simulink library "GOcontroll_Moduline_Target"  (R2023b)
settings: Solver=ode45  StartTime=0.0  StopTime=10.0  RelTol=1e-3  EnableMultiTasking=on
PreLoadFcn:
  | compile_gocontroll_mex;
values from neighbouring files (symbols this model uses):
  id = 2    [sfcn_UDPReceive.m]    (also in sfcn_UDPSend.m = 4)
undefined symbols (not defined in the file or in its folder): C_Cb1Pt10, Cb1Pt10_RAW_ERR_HIGH, Cb1Pt10_RAW_ERR_LOW, Cb1Pt10_SIG_ERR_HIGH, Cb1Pt10_SIG_ERR_LOW, Cb1Pt10_SIG_WAR_HIGH, Cb1Pt10_SIG_WAR_LOW, Pres_0_20_bar_500_4500_mv_inv, signal_x_RAW_ERR_HIGH, signal_x_RAW_ERR_LOW, signal_x_SIG_ERR_HIGH, signal_x_SIG_ERR_LOW, signal_x_SIG_WAR_HIGH, signal_x_SIG_WAR_LOW, signal_x_SPN, Valve1_ACTIVE_DUTY_CYCLE, Valve1_MAX_CURRENT, Valve1_MIN_CURRENT, Valve1_SPN
libraries: $bdroot x17, simulink x12, canmsglib x4
(part 3 of 5)

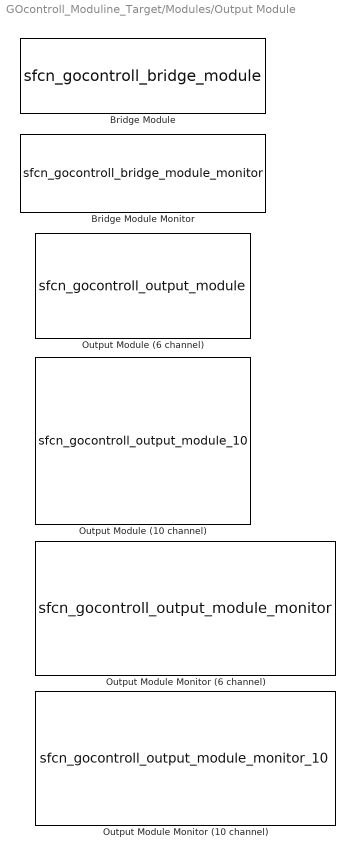
== system GOcontroll_Moduline_Target/Modules/Output Module ==
  Bridge Module : M-S-Function  FunctionName=sfcn_gocontroll_bridge_module  Parameters=tsamp  mask(Bridge Module){tsamp=1, ContrType=GOcontroll Moduline IV, moduleSlot=Moduleslot 1, C1func=Disable (output disabled), C1freq=100 Hz, C2func=Disable (output disabled), C2freq=100 Hz}
      mask prompts: tsamp "Sample time"; ContrType "Controller Type"; moduleSlot "Module Slot"; C1func "Function select"; C1freq "Frequency"; C2func "Function select"; C2freq "Frequency"
      mask help:
      | With this function block, you can configure each output of the bridge module (202001xx). During initialization of the controller, the corresponding outputs of the module are set according the settings. During runtime, the value pushed into the block will control the outputs.
      |
      | Module slot:
      | Sets the location of the module slot where the module is physically
      | plugged into.
      |
      | Channel tabs:
      | Each ouput has its own configuration tab.
      |
      | Function select:
      | Select the desired output configuration.
      |
      | Frequency:
      | In case a duty cycle is used, select the frequency.
      mask init:
      | % array with pinID infos
      | 	moduleSlotInfoStrings = {  	'Module Slot 1',  ...
      | 								'Module Slot 2',  ...
      | 								'Module Slot 3',  ...
      | 								'Module Slot 4',  ...
      | 								'Module Slot 5',  ...
      | 								'Module Slot 6',  ...
      | 								'Module Slot 7',  ...
      | 								'Module Slot 8'};
      | 	% construct the pinID info string
      | 	moduleSlotInfoStr = moduleSlotInfoStrings{moduleSlot};
      | 
      | 
      | 	if(moduleSlot == 1 || moduleSlot == 2)
      | 		connectorId = 'A';
      | 	elseif(moduleSlot == 3 || moduleSlot == 4)
      | 		connectorId = 'B';
      | 	elseif(moduleSlot == 5 || moduleSlot == 6)
      | 		connectorId = 'D';
      | 	else
      | 		connectorId = 'E';
      | 	end
      | 
      | 	if (ContrType == 1) % Moduline IV
      | 		if (mod(moduleSlot,2) == 1) %uneven
      | 			pin1Id = 'Pin 11,12,13';
      | 			pin2Id = 'Pin 17,18,19';
      | 		else
      | 			pin1Id = 'Pin 8,9,10';
      | 			pin2Id = 'Pin 14,15,16';
      | 		end
      | 	elseif(ContrType == 2 || ContrType == 3) % Moduline mini / Moduline display
      | 		if(mod(moduleSlot,2) == 1)
      | 			pin1Id = 'Pin 13,14,15';
      | 			pin2Id = 'Pin 21,22,23';
      | 		else
      | 			pin1Id = 'Pin 10,11,12';
      | 			pin2Id = 'Pin 18,19,20';
      | 		end
      |     end
      |     % register rtw data here because the WriteRTW callback doesn't update
      |     % properly
      |     % Create resource keywords to be reserved in resource database
      | 	modelRTWFields = 	struct('moduleSlot', int2str(moduleSlot),	'C1func', int2str(C1func),'C1freq', int2str(C1freq),...
      | 										'C2func', int2str(C2func),'C2freq', int2str(C2freq));
      | 
      | 	set_param(gcb, 'RTWdata', modelRTWFields);
      mask TypeOptions ContrType: GOcontroll Moduline IV | GOcontroll Moduline Mini | GOcontroll Moduline Display
      mask Callback ContrType:
      | msk = Simulink.Mask.get(gcb);
      | p = msk.getParameter('moduleSlot');
      | 
      | func = get_param(gcb,'ContrType');
      | 
      | if(func == "GOcontroll Moduline IV")
      |     p.TypeOptions = {'Moduleslot 1','Moduleslot 2','Moduleslot 3','Moduleslot 4',...
      |                     'Moduleslot 5','Moduleslot 6','Moduleslot 7','Moduleslot 8'};
      | elseif(func == "GOcontroll Moduline Mini")
      |     p.TypeOptions = {'Moduleslot 1','Moduleslot 2','Moduleslot 3','Moduleslot 4'};
      | elseif (func == "GOcontroll Moduline Display")
      |     p.TypeOptions = {'Moduleslot 1','Moduleslot 2'};
      | end
      mask TypeOptions moduleSlot: Moduleslot 1 | Moduleslot 2 | Moduleslot 3 | Moduleslot 4 | Moduleslot 5 | Moduleslot 6 | Moduleslot 7 | Moduleslot 8
      mask TypeOptions C1func: Disable (output disabled) | Half Bridge duty cycle controlled 0% - 100% duty cycle ( 0 - 1000) | Low side switch  duty cycle controlled 0% - 100% duty cycle (0 - 1000) | High side switch  duty cycle controlled 0% - 100% duty cycle (0 - 1000) | Low side switch On - Off (1-0) | High side switch On - Off (1-0)
      mask TypeOptions C1freq: 100 Hz | 200 Hz | 500 Hz | 1 kHz | 2 kHz | 5 kHz | 10 kHz
      mask TypeOptions C2func: Disable (output disabled) | Half Bridge duty cycle controlled 0% - 100% duty cycle ( 0 - 1000) | Low side switch  duty cycle controlled 0% - 100% duty cycle (0 - 1000) | High side switch  duty cycle controlled 0% - 100% duty cycle (0 - 1000) | Low side switch On - Off (1-0) | High side switch On - Off (1-0)
      mask TypeOptions C2freq: 100 Hz | 200 Hz | 500 Hz | 1 kHz | 2 kHz | 5 kHz | 10 kHz
      mask DialogControl Container4 Prompt: Output 1
      mask DialogControl Container5 Prompt: Output 2
      mask Display:
      | fprintf('Bridge Module\n%s\n\n Controller Connector: %s', moduleSlotInfoStr,connectorId);
      | port_label('input', 1, pin1Id);
      | port_label('input', 2, pin2Id);
      | text(2, 6, ert_linux_target_version());
  Bridge Module Monitor : M-S-Function  FunctionName=sfcn_gocontroll_bridge_module_monitor  Parameters=tsamp  mask(Bridge Module Monitor){tsamp=1, ContrType=GOcontroll Moduline IV, moduleSlot=Moduleslot 1}
      mask prompts: tsamp "Sample time"; ContrType "Controller Type"; moduleSlot "Module Slot"
      mask help:
      | With this function block, you can read parameters from the specified bridge module (202001xx). The block will provide some information about the module such as:
      |
      | Module temperature:
      | The temperature in degrees from the output module.
      |
      | Module ground shift
      | In case the ground connection of the module is poor, the power ground is shifted. The value gives the ground difference in mV and schould be beneath 50 mV
      |
      | Channel current
      | Current related output for each output channel
      mask init:
      | % array with pinID infos
      | 	moduleSlotInfoStrings = {  	'Module slot 1',  ...\
      | 								  'Module slot 2',  ...\
      | 								  'Module slot 3',  ...\
      | 								  'Module slot 4',  ...\
      | 								  'Module slot 5',  ...\
      | 								  'Module slot 6',  ...\
      | 								  'Module slot 7',  ...\
      | 								  'Module slot 8'};
      | 	% construct the pinID info string
      | 	moduleSlotInfoStr = moduleSlotInfoStrings{moduleSlot};
      | 
      | 	if(moduleSlot == 1 || moduleSlot == 2)
      | 		connectorId = 'A';
      | 	elseif(moduleSlot == 3 || moduleSlot == 4)
      | 		connectorId = 'B';
      | 	elseif(moduleSlot == 5 || moduleSlot == 6)
      | 		connectorId = 'D';
      | 	else
      | 		connectorId = 'E';
      | 	end
      | 
      | 	if(ContrType == 1) % Moduline IV
      | 		if(mod(moduleSlot,2) == 1)
      | 			pin1Id = 'Pin 11,12,13';
      | 			pin2Id = 'Pin 17,18,19';
      | 		else
      | 			pin1Id = 'Pin 8,9,10';
      | 			pin2Id = 'Pin 14,15,16';
      | 		end
      | 	elseif(ContrType == 2 || ContrType == 3) % Moduline mini / Moduline display
      | 		if(mod(moduleSlot,2) == 1)
      | 			pin1Id = 'Pin 13,14,15';
      | 			pin2Id = 'Pin 21,22,23';
      | 		else
      | 			pin1Id = 'Pin 10,11,12';
      | 			pin2Id = 'Pin 18,19,20';
      | 		end
      | 	end
      |     % update RTWdata to call WriteRTW again
      | 	modelRTWFields = 	struct('moduleSlot', int2str(moduleSlot));
      | 
      | 	set_param(gcb, 'RTWdata', modelRTWFields);
      mask TypeOptions ContrType: GOcontroll Moduline IV | GOcontroll Moduline Mini | GOcontroll Moduline Display
      mask Callback ContrType:
      | msk = Simulink.Mask.get(gcb);
      |     p = msk.getParameter('moduleSlot');
      |     func = get_param(gcb,'ContrType');
      |     if(func == "GOcontroll Moduline IV")
      |         p.TypeOptions = {'Moduleslot 1','Moduleslot 2','Moduleslot 3','Moduleslot 4',...
      |                         'Moduleslot 5','Moduleslot 6','Moduleslot 7','Moduleslot 8'};
      |     elseif (func == "GOcontroll Moduline Mini")
      |         p.TypeOptions = {'Moduleslot 1','Moduleslot 2','Moduleslot 3','Moduleslot 4'};
      |     elseif (func == "GOcontroll Moduline Display")
      |         p.TypeOptions = {'Moduleslot 1','Moduleslot 2'};
      |     end
      mask TypeOptions moduleSlot: Moduleslot 1 | Moduleslot 2 | Moduleslot 3 | Moduleslot 4 | Moduleslot 5 | Moduleslot 6 | Moduleslot 7 | Moduleslot 8
      mask Display:
      | fprintf('Bridge Module Monitor\n%s\n\n Controller Connector: %s', moduleSlotInfoStr,connectorId);
      | port_label('output', 1, 'Temperature');
      | port_label('output', 2, 'Groundshift');
      | port_label('output', 3, pin1Id);
      | port_label('output', 4, pin2Id);
      | text(2, 6, ert_linux_target_version());
  Output Module (10 channel) : M-S-Function  FunctionName=sfcn_gocontroll_output_module_10  Parameters=tsamp  mask(10 Channel Output Module){tsamp=0.1, ContrType=GOcontroll Moduline IV, moduleSlot=Moduleslot 1, C12freq=200 Hz, C1func=Disable (output disabled), C2func=Disable (output disabled), C34freq=200 Hz, C3func=Disable (output disabled), C4func=Disable (output disabled), C56freq=200 Hz, C5func=Disable (output disabled), C6func=Disable (output disabled), C78freq=200 Hz, C7func=Disable (output disabled), C8func=Disable (output disabled), C910freq=200 Hz, C9func=Disable (output disabled), C10func=Disable (output disabled)}
      mask prompts: tsamp "Sample time"; ContrType "Controller type"; moduleSlot "Module slot"; C12freq "Frequency"; C1func "Channel 1 function"; C2func "Channel 2 function"; C34freq "Frequency"; C3func "Channel 3 function"; C4func "Channel 4 function"; C56freq "Frequency"; C5func "Channel 5 function"; C6func "Channel 6 function"; C78freq "Frequency"; C7func "Channel 7 function"; C8func "Channel 8 function"; C910freq "Frequency"; C9func "Channel 9 function"; C10func "Channel 10 function"
      mask help:
      | With this function block, you can configure each output of the 10 channel output module (202003xx). During initialization of the controller, the corresponding outputs of the module are set according the settings. During runtime, the value pushed into the block will control the outputs.
      |
      | Sample time:
      | Execution frequency from function block. For proper functioning of the output module, use a sampletime of 100 ms or lower.
      |
      | Module slot:
      | Sets the location of the module slot where the module is physically plugged into.
      |
      | Frequency:
      | In case a duty cycle is used, select the frequency.
      |
      | Function select:
      | Select the desired output configuration for each channel
      mask init:
      | % array with pinID infos
      | moduleSlotInfoStrings = {	'Module Slot 1',  ...\
      | 							'Module Slot 2',  ...\
      | 							'Module Slot 3',  ...\
      | 							'Module Slot 4',  ...\
      | 							'Module Slot 5',  ...\
      | 							'Module Slot 6',  ...\
      | 							'Module Slot 7',  ...\
      | 							'Module Slot 8'};
      | % construct the pinID info string
      | moduleSlotInfoStr = moduleSlotInfoStrings{moduleSlot};
      | 
      | if(moduleSlot == 1 || moduleSlot == 2)
      | 	connectorId = 'A';
      | elseif(moduleSlot == 3 || moduleSlot == 4)
      | 	connectorId = 'B';
      | elseif(moduleSlot == 5 || moduleSlot == 6)
      | 	connectorId = 'D';
      | else
      | 	connectorId = 'E';
      | end
      | 
      | if(ContrType == 1) % Moduline IV
      | 	if(moduleSlot == 1 || moduleSlot == 3 || moduleSlot == 5 || moduleSlot == 7)
      | 		pin1Id = 'Pin 13';
      | 		pin2Id = 'Pin 19';
      | 		pin3Id = 'Pin 12';
      | 		pin4Id = 'Pin 18';
      | 		pin5Id = 'Pin 11';
      | 		pin6Id = 'Pin 17';
      | 		pin7Id = 'Pin 25';
      | 		pin8Id = 'Pin 24';
      | 		pin9Id = 'Pin 5';
      | 		pin10Id = 'Pin 4';
      | 	else
      | 		pin1Id = 'Pin 8';
      | 		pin2Id = 'Pin 14';
      | 		pin3Id = 'Pin 9';
      | 		pin4Id = 'Pin 15';
      | 		pin5Id = 'Pin 10';
      | 		pin6Id = 'Pin 16';
      | 		pin7Id = 'Pin 21';
      | 		pin8Id = 'Pin 22';
      | 		pin9Id = 'Pin 3';
      | 		pin10Id = 'Pin 23';
      | 	end
      | elseif(ContrType == 2 || ContrType == 3) % Moduline mini / Moduline display
      | 	if(moduleSlot == 1 || moduleSlot == 3)
      | 		pin1Id = 'Pin 15';
      | 		pin2Id = 'Pin 23';
      | 		pin3Id = 'Pin 14';
      | 		pin4Id = 'Pin 22';
      | 		pin5Id = 'Pin 13';
      | 		pin6Id = 'Pin 21';
      | 		pin7Id = 'Pin 31';
      | 		pin8Id = 'Pin 30';
      | 		pin9Id = 'Pin 5';
      | 		pin10Id = 'Pin 4';
      | 	else
      | 		pin1Id = 'Pin 10';
      | 		pin2Id = 'Pin 18';
      | 		pin3Id = 'Pin 11';
      | 		pin4Id = 'Pin 19';
      | 		pin5Id = 'Pin 12';
      | 		pin6Id = 'Pin 20';
      | 		pin7Id = 'Pin 27';
      | 		pin8Id = 'Pin 28';
      | 		pin9Id = 'Pin 3';
      | 		pin10Id = 'Pin 29';
      | 	end
      | end
      | 
      | % Create resource keywords to be reserved in resource database
      | modelRTWFields = 	struct('moduleSlot', int2str(moduleSlot),	'C12freq', int2str(C12freq),'C1func', int2str(C1func),'C2func', int2str(C2func),...
      | 																'C34freq', int2str(C34freq),'C3func', int2str(C3func),'C4func', int2str(C4func),...
      | 																'C56freq', int2str(C56freq),'C5func', int2str(C5func),'C6func', int2str(C6func),...
      | 																'C78freq', int2str(C78freq),'C7func', int2str(C7func),'C8func', int2str(C8func),...
      | 																'C910freq', int2str(C910freq),'C9func', int2str(C9func),'C10func', int2str(C10func));
      | 
      | set_param(gcb, 'RTWdata', modelRTWFields);
      mask TypeOptions ContrType: GOcontroll Moduline IV | GOcontroll Moduline Mini | GOcontroll Moduline Display
      mask Callback ContrType:
      | msk = Simulink.Mask.get(gcb);
      | p = msk.getParameter('moduleSlot');
      | 
      | func = get_param(gcb,'ContrType');
      | 
      | if(func == "GOcontroll Moduline IV")
      |     p.TypeOptions = {'Moduleslot 1','Moduleslot 2','Moduleslot 3','Moduleslot 4',...
      |                     'Moduleslot 5','Moduleslot 6','Moduleslot 7','Moduleslot 8'};
      | elseif (func == "GOcontroll Moduline Mini")
      |     p.TypeOptions = {'Moduleslot 1','Moduleslot 2','Moduleslot 3','Moduleslot 4'};
      | elseif (func == "GOcontroll Moduline Display")
      |     p.TypeOptions = {'Moduleslot 1','Moduleslot 2'};
      | end
      mask TypeOptions moduleSlot: Moduleslot 1 | Moduleslot 2 | Moduleslot 3 | Moduleslot 4 | Moduleslot 5 | Moduleslot 6 | Moduleslot 7 | Moduleslot 8
      mask TypeOptions C12freq: 100 Hz | 200 Hz
      mask TypeOptions C1func: Disable (output disabled) | High side switch  duty cycle controlled (0 - 1000) | High side switch On - Off (0 - 1)
      mask TypeOptions C2func: Disable (output disabled) | High side switch  duty cycle controlled (0 - 1000) | High side switch On - Off (0 - 1)
      mask TypeOptions C34freq: 100 Hz | 200 Hz
      mask TypeOptions C3func: Disable (output disabled) | High side switch  duty cycle controlled (0 - 1000) | High side switch On - Off (0 - 1)
      mask TypeOptions C4func: Disable (output disabled) | High side switch  duty cycle controlled (0 - 1000) | High side switch On - Off (0 - 1)
      mask TypeOptions C56freq: 100 Hz | 200 Hz
      mask TypeOptions C5func: Disable (output disabled) | High side switch  duty cycle controlled (0 - 1000) | High side switch On - Off (0 - 1)
      mask TypeOptions C6func: Disable (output disabled) | High side switch  duty cycle controlled (0 - 1000) | High side switch On - Off (0 - 1)
      mask TypeOptions C78freq: 100 Hz | 200 Hz
      mask TypeOptions C7func: Disable (output disabled) | High side switch  duty cycle controlled (0 - 1000) | High side switch On - Off (0 - 1)
      mask TypeOptions C8func: Disable (output disabled) | High side switch  duty cycle controlled (0 - 1000) | High side switch On - Off (0 - 1)
      mask TypeOptions C910freq: 100 Hz | 200 Hz
      mask TypeOptions C9func: Disable (output disabled) | High side switch  duty cycle controlled (0 - 1000) | High side switch On - Off (0 - 1)
      mask TypeOptions C10func: Disable (output disabled) | High side switch  duty cycle controlled (0 - 1000) | High side switch On - Off (0 - 1)
      mask DialogControl Container9 Prompt: Output 1 and 2
      mask DialogControl Container12 Prompt: Output 3 and 4
      mask DialogControl Container13 Prompt: Output 5 and 6
      mask DialogControl Container14 Prompt: Output 7 and 8
      mask DialogControl Container15 Prompt: Output 9 and 10
      mask Display:
      | fprintf('10 Channel Output Module\n%s\n\n Controller Connector: %s', moduleSlotInfoStr,connectorId);%%connectorId
      | port_label('input', 1, pin1Id);
      | port_label('input', 2, pin2Id);
      | port_label('input', 3, pin3Id);
      | port_label('input', 4, pin4Id);
      | port_label('input', 5, pin5Id);
      | port_label('input', 6, pin6Id);
      | port_label('input', 7, pin7Id);
      | port_label('input', 8, pin8Id);
      | port_label('input', 9, pin9Id);
      | port_label('input', 10, pin10Id);
      | text(2, 6, ert_linux_target_version());
  Output Module (6 channel) : M-S-Function  FunctionName=sfcn_gocontroll_output_module  Parameters=tsamp  mask(6 Channel Output Module){tsamp=0.1, ContrType=GOcontroll Moduline IV, moduleSlot=Moduleslot 1, C12freq=200 Hz, C1func=Disable (output disabled), C1cur=4000, C1peakCurrent=1000, C1peakTime=500, C2func=Disable (output disabled), C2cur=4000, C2peakCurrent=1000, C2peakTime=500, C34freq=200 Hz, C3func=Disable (output disabled), C3cur=4000, C3peakCurrent=1000, C3peakTime=500, C4func=Disable (output disabled), C4cur=4000, C4peakCurrent=1000, C4peakTime=500, C56freq=200 Hz, C5func=Disable (output disabled), C5cur=4000, C5peakCurrent=1000, C5peakTime=500, C6func=Disable (output disabled), C6cur=4000, C6peakCurrent=1000, C6peakTime=500, C6flmod=Module 1, C6flchan=Channel 1, C6flgain=100, C6flbasicDuty=0}
      mask prompts: tsamp "Sample time"; ContrType "Controller Type"; moduleSlot "Module slot"; C12freq "Frequency"; C1func "Channel 1 function"; C1cur "Channel 1 Imax [mA]"; C1peakCurrent "Peak Current [mA]"; C1peakTime "Peak time [ms]"; C2func "Channel 2 function"; C2cur "Channel 2 Imax [mA]"; C2peakCurrent "Peak Current [mA]"; C2peakTime "Peak time [ms]"; C34freq "Frequency"; C3func "Channel 3 function"; C3cur "Channel 3 Imax [mA]"; C3peakCurrent "Peak Current [mA]"; C3peakTime "Peak time [ms]"; C4func "Channel 4 function"; C4cur "Channel 4 Imax [mA]"; C4peakCurrent "Peak Current [mA]"; C4peakTime "Peak time [ms]"; C56freq "Frequency"; C5func "Channel 5 function"; C5cur "Channel 5 Imax [mA]"; C5peakCurrent "Peak Current [mA]"; C5peakTime "Peak time [ms]"; C6func "Channel 6 function"; C6cur "Channel 6 Imax [mA]"; C6peakCurrent "Peak Current [mA]"; C6peakTime "Peak time [ms]"; C6flmod "Reference signal module"; C6flchan "Reference signal channel"; C6flgain "Fast loop gain (x100)"; C6flbasicDuty "Fast loop basic duty (0-1000)"
      mask help:
      | With this block, you can configure each output of the 6 channel output module (202002xx). During initialization of the controller, the corresponding outputs of the module are set according the settings. During runtime, the value pushed into the block will control the outputs.
      |
      | Sample time:
      | Execution frequency from function block. For proper functioning of the output module, us a sampletime of 100 ms or lower.
      |
      | Module slot:
      | Sets the location of the module slot where the module is physically plugged into.
      |
      | Frequency:
      | In case a duty cycle is used, select the frequency.
      |
      | Function select:
      | Select the desired output configuration for each channel
      mask init:
      | % array with pinID infos
      | moduleSlotInfoStrings = {	'Module slot 1',  ...\
      | 							'Module slot 2',  ...\
      | 							'Module slot 3',  ...\
      | 							'Module slot 4',  ...\
      | 							'Module slot 5',  ...\
      | 							'Module slot 6',  ...\
      | 							'Module slot 7',  ...\
      | 							'Module slot 8'};
      | % construct the pinID info string
      | moduleSlotInfoStr = moduleSlotInfoStrings{moduleSlot};
      | 
      | if(moduleSlot == 1 || moduleSlot == 2)
      | 	connectorId = 'A';
      | elseif(moduleSlot == 3 || moduleSlot == 4)
      | 	connectorId = 'B';
      | elseif(moduleSlot == 5 || moduleSlot == 6)
      | 	connectorId = 'D';
      | else
      | 	connectorId = 'E';
      | end
      | 
      | if(ContrType == 1) % Moduline IV
      | 	if(moduleSlot == 1 || moduleSlot == 3 || moduleSlot == 5 || moduleSlot == 7)
      | 		pin1Id = 'Pin 13';
      | 		pin2Id = 'Pin 19';
      | 		pin3Id = 'Pin 12';
      | 		pin4Id = 'Pin 18';
      | 		pin5Id = 'Pin 11';
      | 		pin6Id = 'Pin 17';
      | 	else
      | 		pin1Id = 'Pin 8';
      | 		pin2Id = 'Pin 14';
      | 		pin3Id = 'Pin 9';
      | 		pin4Id = 'Pin 15';
      | 		pin5Id = 'Pin 10';
      | 		pin6Id = 'Pin 16';
      | 	end
      | elseif(ContrType == 2 || ContrType == 3) % Moduline mini / Moduline Display
      | 	if(moduleSlot == 1 || moduleSlot == 3)
      | 		pin1Id = 'Pin 15';
      | 		pin2Id = 'Pin 23';
      | 		pin3Id = 'Pin 14';
      | 		pin4Id = 'Pin 22';
      | 		pin5Id = 'Pin 13';
      | 		pin6Id = 'Pin 21';
      | 	else
      | 		pin1Id = 'Pin 10';
      | 		pin2Id = 'Pin 18';
      | 		pin3Id = 'Pin 11';
      | 		pin4Id = 'Pin 19';
      | 		pin5Id = 'Pin 12';
      | 		pin6Id = 'Pin 20';
      | 	end
      | end
      | 
      | % Create resource keywords to be reserved in resource database
      | modelRTWFields = 	struct('moduleSlot', int2str(moduleSlot),	'C12freq', int2str(C12freq),...
      | 																'C1func', int2str(C1func),'C2func', int2str(C2func),...
      | 																'C34freq', int2str(C34freq),...
      | 																'C3func', int2str(C3func),'C4func', int2str(C4func),...
      | 																'C56freq', int2str(C56freq),...
      | 																'C5func', int2str(C5func),'C6func', int2str(C6func),...
      | 																'C1cur', int2str(C1cur),'C2cur', int2str(C2cur),...
      | 																'C3cur', int2str(C3cur),'C4cur', int2str(C4cur),...
      | 																'C5cur', int2str(C5cur),'C6cur', int2str(C6cur),...
      | 																'C1peakCurrent', int2str(C1peakCurrent),'C1peakTime', int2str(C1peakTime),...
      | 																'C2peakCurrent', int2str(C2peakCurrent),'C2peakTime', int2str(C2peakTime),...
      | 																'C3peakCurrent', int2str(C3peakCurrent),'C3peakTime', int2str(C3peakTime),...
      | 																'C4peakCurrent', int2str(C4peakCurrent),'C4peakTime', int2str(C4peakTime),...
      | 																'C5peakCurrent', int2str(C5peakCurrent),'C5peakTime', int2str(C5peakTime),...
      | 																'C6peakCurrent', int2str(C6peakCurrent),'C6peakTime', int2str(C6peakTime),...
      |                                                                 'C6flmod', int2str(C6flmod),'C6flchan', int2str(C6flchan),...
      | 																'C6flgain',int2str(C6flgain), 'C6flbasicDuty', int2str(C6flbasicDuty));
      | 
      | set_param(gcb, 'RTWdata', modelRTWFields);
      mask TypeOptions ContrType: GOcontroll Moduline IV | GOcontroll Moduline Mini | GOcontroll Moduline Display
      mask Callback ContrType:
      | msk = Simulink.Mask.get(gcb);
      | p = msk.getParameter('moduleSlot');
      | refslot = msk.getParameter('C6flmod');
      | 
      | func = get_param(gcb,'ContrType');
      | MIVTypeOptions = {'Moduleslot 1','Moduleslot 2','Moduleslot 3','Moduleslot 4',...
      |                     'Moduleslot 5','Moduleslot 6','Moduleslot 7','Moduleslot 8'};
      | MMiniTypeOptions = {'Moduleslot 1','Moduleslot 2','Moduleslot 3','Moduleslot 4'};
      | MDisplayTypeOptions = {'Moduleslot 1','Moduleslot 2'};
      | 
      | if(func == "GOcontroll Moduline IV")
      |     p.TypeOptions = MIVTypeOptions;
      |     refslot.TypeOptions = MIVTypeOptions;
      | elseif(func == "GOcontroll Moduline Mini")
      |     p.TypeOptions = MMiniTypeOptions;
      |     refslot.TypeOptions = MMiniTypeOptions;
      | elseif (func == "GOcontroll Moduline Display")
      |     p.TypeOptions = MDisplayTypeOptions;
      |     refslot.TypeOptions = MDisplayTypeOptions;
      | end
      mask TypeOptions moduleSlot: Moduleslot 1 | Moduleslot 2 | Moduleslot 3 | Moduleslot 4 | Moduleslot 5 | Moduleslot 6 | Moduleslot 7 | Moduleslot 8
      mask TypeOptions C12freq: 100 Hz | 200 Hz | 500 Hz | 1 kHz | 2 kHz | 5 kHz | 10 kHz
      mask TypeOptions C1func: Disable (output disabled) | Half Bridge duty cycle controlled (0 - 1000) | Low side switch  duty cycle controlled (0 - 1000) | High side switch  duty cycle controlled (0 - 1000) | Low side switch On - Off (0 - 1) | High side switch On - Off (0 - 1) | Peak and hold current mode (Half Bridge) | Frequency output 0 - 500 Hz (0-500)
      mask Callback C1func:
      | func = get_param(gcb,'C1func');
      | p=Simulink.Mask.get(gcb);
      | a=p.getParameter('C1peakCurrent');
      | b=p.getParameter('C1peakTime');
      | c=p.getParameter('C1cur');
      | 
      | if( func == "Peak and hold current mode (Half Bridge)")
      | a.set('Visible','on');
      | b.set('Visible','on');
      | else
      | a.set('Visible','off');
      | b.set('Visible','off');
      | end
      | 
      | if( func == "Disable (output disabled)")
      | c.set('Enabled','off');
      | else
      | c.set('Enabled','on');
      | end
      mask TypeOptions C2func: Disable (output disabled) | Half Bridge duty cycle controlled (0 - 1000) | Low side switch  duty cycle controlled (0 - 1000) | High side switch  duty cycle controlled (0 - 1000) | Low side switch On - Off (0 - 1) | High side switch On - Off (0 - 1) | Peak and hold current mode (Half Bridge) | Frequency output 0 - 500 Hz (0-500)
      mask Callback C2func:
      | func = get_param(gcb,'C2func');
      | p=Simulink.Mask.get(gcb);
      | a=p.getParameter('C2peakCurrent');
      | b=p.getParameter('C2peakTime');
      | c=p.getParameter('C2cur');
      | 
      | if( func == "Peak and hold current mode (Half Bridge)")
      | a.set('Visible','on');
      | b.set('Visible','on');
      | else
      | a.set('Visible','off');
      | b.set('Visible','off');
      | end
      | 
      | if( func == "Disable (output disabled)")
      | c.set('Enabled','off');
      | else
      | c.set('Enabled','on');
      | end
      mask TypeOptions C34freq: 100 Hz | 200 Hz | 500 Hz | 1 kHz | 2 kHz | 5 kHz | 10 kHz
      mask TypeOptions C3func: Disable (output disabled) | Half Bridge duty cycle controlled (0 - 1000) | Low side switch  duty cycle controlled (0 - 1000) | High side switch  duty cycle controlled (0 - 1000) | Low side switch On - Off (0 - 1) | High side switch On - Off (0 - 1) | Peak and hold current mode (Half Bridge) | Frequency output 0 - 500 Hz (0-500)
      mask Callback C3func:
      | func = get_param(gcb,'C3func');
      | p=Simulink.Mask.get(gcb);
      | a=p.getParameter('C3peakCurrent');
      | b=p.getParameter('C3peakTime');
      | c=p.getParameter('C3cur');
      | 
      | if( func == "Peak and hold current mode (Half Bridge)")
      | a.set('Visible','on');
      | b.set('Visible','on');
      | else
      | a.set('Visible','off');
      | b.set('Visible','off');
      | end
      | 
      | if( func == "Disable (output disabled)")
      | c.set('Enabled','off');
      | else
      | c.set('Enabled','on');
      | end
      mask TypeOptions C4func: Disable (output disabled) | Half Bridge duty cycle controlled (0 - 1000) | Low side switch  duty cycle controlled (0 - 1000) | High side switch  duty cycle controlled (0 - 1000) | Low side switch On - Off (0 - 1) | High side switch On - Off (0 - 1) | Peak and hold current mode (Half Bridge) | Frequency output 0 - 500 Hz (0-500)
      mask Callback C4func:
      | func = get_param(gcb,'C4func');
      | p=Simulink.Mask.get(gcb);
      | a=p.getParameter('C4peakCurrent');
      | b=p.getParameter('C4peakTime');
      | c=p.getParameter('C4cur');
      | 
      | if( func == "Peak and hold current mode (Half Bridge)")
      | a.set('Visible','on');
      | b.set('Visible','on');
      | else
      | a.set('Visible','off');
      | b.set('Visible','off');
      | end
      | 
      | if( func == "Disable (output disabled)")
      | c.set('Enabled','off');
      | else
      | c.set('Enabled','on');
      | end
      mask TypeOptions C56freq: 100 Hz | 200 Hz | 500 Hz | 1 kHz | 2 kHz | 5 kHz | 10 kHz
      mask TypeOptions C5func: Disable (output disabled) | Half Bridge duty cycle controlled (0 - 1000) | Low side switch  duty cycle controlled (0 - 1000) | High side switch  duty cycle controlled (0 - 1000) | Low side switch On - Off (0 - 1) | High side switch On - Off (0 - 1) | Peak and hold current mode (Half Bridge) | Frequency output 0 - 500 Hz (0-500)
      mask Callback C5func:
      | func = get_param(gcb,'C5func');
      | p=Simulink.Mask.get(gcb);
      | a=p.getParameter('C5peakCurrent');
      | b=p.getParameter('C5peakTime');
      | c=p.getParameter('C5cur');
      | 
      | if( func == "Peak and hold current mode (Half Bridge)")
      | a.set('Visible','on');
      | b.set('Visible','on');
      | else
      | a.set('Visible','off');
      | b.set('Visible','off');
      | end
      | 
      | if( func == "Disable (output disabled)")
      | c.set('Enabled','off');
      | else
      | c.set('Enabled','on');
      | end
      mask TypeOptions C6func: Disable (output disabled) | Half Bridge duty cycle controlled (0 - 1000) | Low side switch  duty cycle controlled (0 - 1000) | High side switch  duty cycle controlled (0 - 1000) | Low side switch On - Off (0 - 1) | High side switch On - Off (0 - 1) | Peak and hold current mode (Half Bridge) | Frequency output 0 - 500 Hz (0-500) | Fast loop half bridge control
      mask Callback C6func:
      | func = get_param(gcb,'C6func');
      | p=Simulink.Mask.get(gcb);
      | pc=p.getParameter('C6peakCurrent');
      | pt=p.getParameter('C6peakTime');
      | c=p.getParameter('C6cur');
      | flm=p.getParameter('C6flmod');
      | flc=p.getParameter('C6flchan');
      | flg=p.getParameter('C6flgain');
      | flbd=p.getParameter('C6flbasicDuty');
      | 
      | if( func == "Peak and hold current mode (Half Bridge)")
      | pc.set('Visible','on');
      | pt.set('Visible','on');
      | else
      | pc.set('Visible','off');
      | pt.set('Visible','off');
      | end
      | 
      | if( func == "Fast loop half bridge control")
      |     flm.set('Visible', 'on');
      |     flc.set('Visible', 'on');
      |     flg.set('Visible', 'on');
      |     flbd.set('Visible', 'on');
      | else
      |     flm.set('Visible', 'off');
      |     flc.set('Visible', 'off');
      |     flg.set('Visible', 'off');
      |     flbd.set('Visible', 'off');
      | end
      | 
      | if( func == "Disable (output disabled)")
      | c.set('Enabled','off');
      | else
      | c.set('Enabled','on');
      | end
      mask TypeOptions C6flmod: Module 1 | Module 2 | Module 3 | Module 4 | Module 5 | Module 6 | Module 7 | Module 8
      mask TypeOptions C6flchan: Channel 1 | Channel 2 | Channel 3 | Channel 4 | Channel 5 | Channel 6
      mask DialogControl Container9 Prompt: Output 1 and 2
      mask DialogControl Container12 Prompt: Output 3 and 4
      mask DialogControl Container13 Prompt: Output 5 and 6
      mask Display:
      | fprintf('6 Channel Output Module\n%s\n\n Controller Connector: %s', moduleSlotInfoStr,connectorId);%%connectorId
      | port_label('input', 1, pin1Id);
      | port_label('input', 2, pin2Id);
      | port_label('input', 3, pin3Id);
      | port_label('input', 4, pin4Id);
      | port_label('input', 5, pin5Id);
      | port_label('input', 6, pin6Id);
      | text(2, 6, ert_linux_target_version());
  Output Module Monitor (10 channel) : M-S-Function  FunctionName=sfcn_gocontroll_output_module_monitor_10  Parameters=tsamp, moduleSlot  mask(Output Module Monitor (10 channel)){tsamp=0.1, ContrType=GOcontroll Moduline IV, moduleSlot=Moduleslot 1}
      mask prompts: tsamp "Sample time"; ContrType "Controller Type"; moduleSlot "Module Slot"
      mask help:
      | With this function block, you can read parameters from the specified 10 channel output module (202003xx). The block will provide some information about the module such as:
      |
      | Module temperature:
      | The temperature in degrees from the output module.
      |
      | Module ground shift
      | In case the ground connection of the module is poor, the power ground is shifted. The value gives the ground difference in mV and schould be beneath 50 mV
      |
      | Module supply voltage
      | The measured supply voltage of the module in mV.
      |
      | Module error code
      | If the module encounters an error, the relevant fault bit will be set here. See the software manual on the website: https://gocontroll.com/downloads/
      |
      | Module current
      | The total current of the module is measured and given in mA.
      mask init:
      | % array with pinID infos
      | moduleSlotInfoStrings = {	'Module slot 1',  ...\
      | 							'Module slot 2',  ...\
      | 							'Module slot 3',  ...\
      | 							'Module slot 4',  ...\
      | 							'Module slot 5',  ...\
      | 							'Module slot 6',  ...\
      | 							'Module slot 7',  ...\
      | 							'Module slot 8'};
      | % construct the pinID info string
      | moduleSlotInfoStr = moduleSlotInfoStrings{moduleSlot};
      | 
      | if(moduleSlot == 1 || moduleSlot == 2)
      | connectorId = 'A';
      | elseif(moduleSlot == 3 || moduleSlot == 4)
      | connectorId = 'B';
      | elseif(moduleSlot == 5 || moduleSlot == 6)
      | connectorId = 'D';
      | else
      | connectorId = 'E';
      | end
      | 
      | % Create resource keywords to be reserved in resource database
      | modelRTWFields = struct('moduleSlot', int2str(moduleSlot));
      | 
      | set_param(gcb, 'RTWdata', modelRTWFields);
      mask TypeOptions ContrType: GOcontroll Moduline IV | GOcontroll Moduline Mini | GOcontroll Moduline Display
      mask Callback ContrType:
      | msk = Simulink.Mask.get(gcb);
      | p = msk.getParameter('moduleSlot');
      | 
      | func = get_param(gcb,'ContrType');
      | 
      | if(func == "GOcontroll Moduline IV")
      |     p.TypeOptions = {'Moduleslot 1','Moduleslot 2','Moduleslot 3','Moduleslot 4',...
      |                     'Moduleslot 5','Moduleslot 6','Moduleslot 7','Moduleslot 8'};
      | elseif (func == "GOcontroll Moduline Mini")
      |     p.TypeOptions = {'Moduleslot 1','Moduleslot 2','Moduleslot 3','Moduleslot 4'};
      | elseif (func == "GOcontroll Moduline Display")
      |     p.TypeOptions = {'Moduleslot 1','Moduleslot 2'};
      | end
      mask TypeOptions moduleSlot: Moduleslot 1 | Moduleslot 2 | Moduleslot 3 | Moduleslot 4 | Moduleslot 5 | Moduleslot 6 | Moduleslot 7 | Moduleslot 8
      mask Display:
      | fprintf('10 Channel Output Module Monitor\n%s\n\n Controller Connector: %s', moduleSlotInfoStr,connectorId);
      | port_label('output', 1, 'Temperature');
      | port_label('output', 2, 'Ground');
      | port_label('output', 3, 'Supply');
      | port_label('output', 4, 'Status');
      | port_label('output', 5, "Current");
      | 
      | 
      | text(2, 6, ert_linux_target_version());
  Output Module Monitor (6 channel) : M-S-Function  FunctionName=sfcn_gocontroll_output_module_monitor  Parameters=tsamp, moduleSlot, C1duty, C2duty, C3duty, C4duty, C5duty, C6duty  mask(Output Module Monitor){tsamp=0.1, ContrType=GOcontroll Moduline IV, moduleSlot=Moduleslot 1, C1duty=0, C2duty=0, C3duty=0, C4duty=0, C5duty=0, C6duty=0}
      mask prompts: tsamp "Sample time"; ContrType "Controller Type"; moduleSlot "Module Slot"
      mask help:
      | With this function block, you can read parameters from the specified 6 channel output module (202002xx). The block will provide some information about the module such as:
      |
      | Module temperature:
      | The temperature in degrees from the output module.
      |
      | Module ground shift
      | In case the ground connection of the module is poor, the power ground is shifted. The value gives the ground difference in mV and schould be beneath 50 mV
      |
      | Module supply voltage
      | The measured supply voltage of the module in mV. This output only works for hardware version 7 and above, gives off 0 otherwise.
      |
      | Channel current
      | The current from each channel is measured and given in mA. If the ouput is configured as high side, the result will be positive. If the ouput is configured as low side, the value will be negative
      |
      | Channel duty cycle
      | This output only appears if the corresponding output module block has a channel in peak and hold mode, and it only works for module firmware 2.1.0 and higher.
      | This output can be used to monitor the actual output duty cycle. This value can then be used to perform extra checks on the output in this mode.
      mask init:
      | % array with pinID infos
      | moduleSlotInfoStrings = {	'Module slot 1',  ...\
      | 							'Module slot 2',  ...\
      | 							'Module slot 3',  ...\
      | 							'Module slot 4',  ...\
      | 							'Module slot 5',  ...\
      | 							'Module slot 6',  ...\
      | 							'Module slot 7',  ...\
      | 							'Module slot 8'};
      | % construct the pinID info string
      | moduleSlotInfoStr = moduleSlotInfoStrings{moduleSlot};
      | 
      | if(moduleSlot == 1 || moduleSlot == 2)
      | connectorId = 'A';
      | elseif(moduleSlot == 3 || moduleSlot == 4)
      | connectorId = 'B';
      | elseif(moduleSlot == 5 || moduleSlot == 6)
      | connectorId = 'D';
      | else
      | connectorId = 'E';
      | end
      | 
      | if(ContrType == 1) % Moduline IV
      | 	if(moduleSlot == 1 || moduleSlot == 3 || moduleSlot == 5 || moduleSlot == 7)
      | 		pin1Id = 'Pin 13';
      | 		pin2Id = 'Pin 19';
      | 		pin3Id = 'Pin 12';
      | 		pin4Id = 'Pin 18';
      | 		pin5Id = 'Pin 11';
      | 		pin6Id = 'Pin 17';
      | 	else
      | 		pin1Id = 'Pin 8';
      | 		pin2Id = 'Pin 14';
      | 		pin3Id = 'Pin 9';
      | 		pin4Id = 'Pin 15';
      | 		pin5Id = 'Pin 10';
      | 		pin6Id = 'Pin 16';
      | 	end
      | elseif(ContrType == 2 || ContrType == 3) % Moduline mini / Moduline display
      | 	if(moduleSlot == 1 || moduleSlot == 3)
      | 		pin1Id = 'Pin 15';
      | 		pin2Id = 'Pin 23';
      | 		pin3Id = 'Pin 14';
      | 		pin4Id = 'Pin 22';
      | 		pin5Id = 'Pin 13';
      | 		pin6Id = 'Pin 17';
      | 	else
      | 		pin1Id = 'Pin 10';
      | 		pin2Id = 'Pin 18';
      | 		pin3Id = 'Pin 11';
      | 		pin4Id = 'Pin 19';
      | 		pin5Id = 'Pin 12';
      | 		pin6Id = 'Pin 20';
      | 	end
      | end
      | 
      | 
      | 
      | % Create resource keywords to be reserved in resource database
      | modelRTWFields = 	struct('moduleSlot', int2str(moduleSlot), 'C1duty', int2str(C1duty), 'C2duty', int2str(C2duty), ...
      |     'C3duty', int2str(C3duty), 'C4duty', int2str(C4duty), 'C5duty', int2str(C5duty), 'C6duty', int2str(C6duty));
      | 
      | set_param(gcb, 'RTWdata', modelRTWFields);
      mask TypeOptions ContrType: GOcontroll Moduline IV | GOcontroll Moduline Mini | GOcontroll Moduline Display
      mask Callback ContrType:
      | msk = Simulink.Mask.get(gcb);
      | p = msk.getParameter('moduleSlot');
      | 
      | func = get_param(gcb,'ContrType');
      | 
      | if(func == "GOcontroll Moduline IV")
      |     p.TypeOptions = {'Moduleslot 1','Moduleslot 2','Moduleslot 3','Moduleslot 4',...
      |                     'Moduleslot 5','Moduleslot 6','Moduleslot 7','Moduleslot 8'};
      | elseif (func == "GOcontroll Moduline Mini")
      |     p.TypeOptions = {'Moduleslot 1','Moduleslot 2','Moduleslot 3','Moduleslot 4'};
      | elseif (func == "GOcontroll Moduline Display")
      |     p.TypeOptions = {'Moduleslot 1','Moduleslot 2'};
      | end
      mask TypeOptions moduleSlot: Moduleslot 1 | Moduleslot 2 | Moduleslot 3 | Moduleslot 4 | Moduleslot 5 | Moduleslot 6 | Moduleslot 7 | Moduleslot 8
      mask Callback moduleSlot:
      | moduleSlot = get_param(gcb, 'moduleSlot');
      | blockPath = split(gcb, '/');
      | output_modules = find_system(blockPath(1), 'RegExp', 'on', 'FollowLinks', 'on', 'MaskType', '6 Channel Output Module');
      | for idx = 1:length(output_modules)
      |     if char(get_param(output_modules, 'moduleSlot')) == char(moduleSlot)
      |         for jdx = 1:6
      |             if get_param(output_modules, sprintf('C%dfunc',jdx)) == "Peak and hold current mode (Half Bridge)"
      |                 set_param(gcb, sprintf('C%dduty',jdx), "1");
      |             else
      |                 set_param(gcb, sprintf('C%dduty',jdx), "0");
      |             end
      |         end
      |         break
      |     else
      |         for jdx = 1:6
      |             set_param(gcb, sprintf('C%dduty',jdx), "0");
      |         end
      |     end
      | end
      mask Display:
      | fprintf('6 Channel Output Module Monitor\n%s\n\n Controller Connector: %s', moduleSlotInfoStr,connectorId);
      | port_label('output', 1, 'Temperature');
      | port_label('output', 2, 'Ground');
      | port_label('output', 3, 'Supply');
      | port_label('output', 4, 'Status');
      | pinIdx = 5;
      | port_label('output', pinIdx, strcat(pin1Id, " current"));
      | pinIdx = pinIdx + 1;
      | if C1duty == 1
      |     port_label('output', pinIdx, strcat(pin1Id, " duty cycle"));
      |     pinIdx = pinIdx + 1;
      | end
      | 
      | port_label('output', pinIdx, strcat(pin2Id, " current"));
      | pinIdx = pinIdx + 1;
      | if C2duty == 1
      |     port_label('output', pinIdx, strcat(pin2Id, " duty cycle"));
      |     pinIdx = pinIdx + 1;
      | end
      | 
      | port_label('output', pinIdx, strcat(pin3Id, " current"));
      | pinIdx = pinIdx + 1;
      | if C3duty == 1
      |     port_label('output', pinIdx, strcat(pin3Id, " duty cycle"));
      |     pinIdx = pinIdx + 1;
      | end
      | 
      | port_label('output', pinIdx, strcat(pin4Id, " current"));
      | pinIdx = pinIdx + 1;
      | if C4duty == 1
      |     port_label('output', pinIdx, strcat(pin4Id, " duty cycle"));
      |     pinIdx = pinIdx + 1;
      | end
      | 
      | port_label('output', pinIdx, strcat(pin5Id, " current"));
      | pinIdx = pinIdx + 1;
      | if C5duty == 1
      |     port_label('output', pinIdx, strcat(pin5Id, " duty cycle"));
      |     pinIdx = pinIdx + 1;
      | end
      | 
      | port_label('output', pinIdx, strcat(pin6Id, " current"));
      | pinIdx = pinIdx + 1;
      | if C6duty == 1
      |     port_label('output', pinIdx, strcat(pin6Id, " duty cycle"));
      |     pinIdx = pinIdx + 1;
      | end
      | 
      | text(2, 6, ert_linux_target_version());

== system GOcontroll_Moduline_Target/Network/MQTT ==
